simulink model "simulation_input_constraint"  (R2023b)
settings: Solver=VariableStepAuto  StartTime=0  StopTime=t_end  RelTol=1e-3
InitFcn:
  | param = plant_param();
values from neighbouring files (symbols this model uses):
  t_end = (N-1)*Ts    [plot_bode.m]
libraries: fl_lib x8, nesl_utility x7, simulink x1
(part 3 of 3)

== matlab function simulation_input_constraint/Subsystem/MATLAB Function ==
  data: Ps input; ub output; P input; param parameter
function ub = inflow(Ps,P,param)
    ub = input_constraint(Ps,P,param);
end

== matlab function simulation_input_constraint/Subsystem/MATLAB Function1 ==
  data: P input; ub output; Pa input; param parameter
function ub = outflow(P,Pa,param)
    ub = input_constraint(P,Pa,param);
end
